simulink model "CubeSatTEST"  (R2024b)
settings: Solver=ode4  StartTime=simul.t0  StopTime=simul.tf  FixedStep=0.01  RelTol=1e-3
values from neighbouring files (symbols this model uses):
  alpha1 = 0.7    [mainSimTEST.m]
  alpha2 = 0.3    [mainSimTEST.m]
undefined symbols (not defined in the file or in its folder): act, DiscIntNeverNeededParam, env, flag, IC, K, orb, sat, sens
libraries: matrix_library x55, simulink_extras x5, simulink x2
(part 2 of 10)

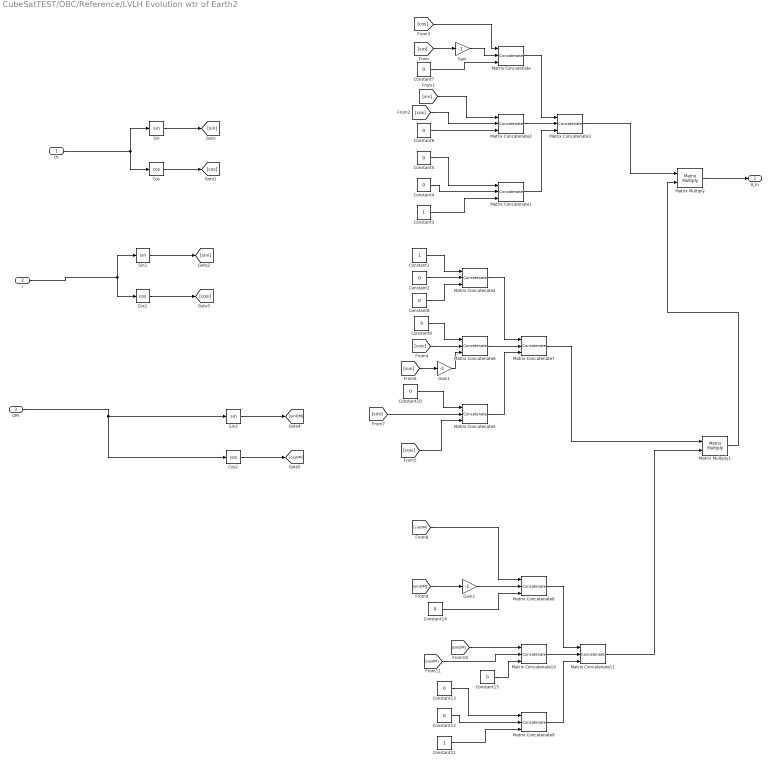
== system CubeSatTEST/OBC/Reference/LVLH Evolution wtr of Earth2 ==
  th : Inport
  i : Inport  Port=2
  OM : Inport  Port=3
  Constant1 : Constant
  Constant{2,4..10,12..15} (12 alike) : Constant  Value=0
  Constant11 : Constant
  Constant3 : Constant
  Cos : Trigonometry  Operator=cos
  Cos1 : Trigonometry  Operator=cos
  Cos2 : Trigonometry  Operator=cos
  Gain : Gain  Gain=-1
  Gain1 : Gain  Gain=-1
  Gain2 : Gain  Gain=-1
  Matrix Concatenate{,1..2,4..6,8..10} (9 alike) : Concatenate  NumInputs=3  Mode=Multidimensional array
  Matrix Concatenate11 : Concatenate  NumInputs=3  Mode=Multidimensional array  ConcatenateDimension=2
  Matrix Concatenate3 : Concatenate  NumInputs=3  Mode=Multidimensional array  ConcatenateDimension=2
  Matrix Concatenate7 : Concatenate  NumInputs=3  Mode=Multidimensional array  ConcatenateDimension=2
  Matrix Multiply : Product  Multiplication=Matrix(*)
  Matrix Multiply1 : Product  Multiplication=Matrix(*)
  Sin : Trigonometry
  Sin1 : Trigonometry
  Sin2 : Trigonometry
  A_ln : Outport
  wires:
  Cos/1 -> [cos]
  Matrix Concatenate1/1 -> Matrix Concatenate3/3
  th/1 -> Cos/1, Sin/1
  Matrix Concatenate/1 -> Matrix Concatenate3/1
  Constant5/1 -> Matrix Concatenate1/1
  Constant3/1 -> Matrix Concatenate1/3
  [cos] -> Matrix Concatenate/1
  Sin/1 -> [sin]
  Constant6/1 -> Matrix Concatenate2/3
  Constant7/1 -> Matrix Concatenate/3
  Constant4/1 -> Matrix Concatenate1/2
  Matrix Concatenate2/1 -> Matrix Concatenate3/2
  [cos] -> Matrix Concatenate2/2
  [sin] -> Matrix Concatenate2/1
  Gain/1 -> Matrix Concatenate/2
  [sin] -> Gain/1
  Cos1/1 -> [cosi]
  Sin1/1 -> [sini]
  i/1 -> Cos1/1, Sin1/1
  Matrix Multiply/1 -> A_ln/1
  Matrix Concatenate3/1 -> Matrix Multiply/1
  Matrix Concatenate6/1 -> Matrix Concatenate7/2
  Matrix Concatenate5/1 -> Matrix Concatenate7/3
  Matrix Concatenate4/1 -> Matrix Concatenate7/1
  Constant1/1 -> Matrix Concatenate4/1
  Constant2/1 -> Matrix Concatenate4/2
  Constant8/1 -> Matrix Concatenate4/3
  Constant9/1 -> Matrix Concatenate6/1
  Constant10/1 -> Matrix Concatenate5/1
  [cosi] -> Matrix Concatenate5/3
  [cosi] -> Matrix Concatenate6/2
  [sini] -> Matrix Concatenate5/2
  [sini] -> Gain1/1
  Gain1/1 -> Matrix Concatenate6/3
  Matrix Multiply1/1 -> Matrix Multiply/2
  Matrix Concatenate7/1 -> Matrix Multiply1/1
  OM/1 -> Cos2/1, Sin2/1
  Cos2/1 -> [cosOM]
  Sin2/1 -> [sinOM]
  Matrix Concatenate10/1 -> Matrix Concatenate11/2
  Matrix Concatenate9/1 -> Matrix Concatenate11/3
  Matrix Concatenate8/1 -> Matrix Concatenate11/1
  Matrix Concatenate11/1 -> Matrix Multiply1/2
  Constant13/1 -> Matrix Concatenate9/1
  Constant11/1 -> Matrix Concatenate9/3
  Constant12/1 -> Matrix Concatenate9/2
  Gain2/1 -> Matrix Concatenate8/2
  Constant14/1 -> Matrix Concatenate8/3
  [cosOM] -> Matrix Concatenate8/1
  [sinOM] -> Gain2/1
  [sinOM] -> Matrix Concatenate10/1
  [cosOM] -> Matrix Concatenate10/2
  Constant15/1 -> Matrix Concatenate10/3

== system CubeSatTEST/OBC/Reference/Magnetic Field order 1 ==
  Vector : Inport
  Clock : Clock
  Constant : Constant  Value=env.mag.dgrf2020
  Constant1 : Constant  Value=env.Earth.R
  Constant2 : Constant  Value=3
  Constant3 : Constant  Value=env.Earth.magInclination
  Constant4 : Constant  Value=3
  Cos : Trigonometry  Operator=cos
  Cos1 : Trigonometry  Operator=cos
  Divide : Product  Inputs=***/
  Divide1 : Product  Inputs=*/
  Divide2 : Product  Inputs=*/
  Dot Product : DotProduct  OutDataTypeStr=Inherit: Inherit via internal rule
  Gain : Gain  Gain=3
  Gain1 : Gain  Gain=env.Earth.omega
  Mux : Mux  Inputs=3
  Norm : Subsystem
  Norm1 : Subsystem
  Norm2 : Subsystem
  Power : Math  Operator=pow
  Power1 : Math  Operator=pow
  Product : Product
  Product1 : Product
  Product2 : Product
  Sin : Trigonometry
  Sin1 : Trigonometry
  Sqrt : Sqrt
  Square : Math  Operator=square
  Subtract : Sum  Inputs=+-
  Sum of Elements : Sum  Inputs=+
  B_n : Outport
  wires:
  Constant/1 -> Square/1
  Square/1 -> Sum of Elements/1
  Sum of Elements/1 -> Sqrt/1
  Constant1/1 -> Power/1
  Constant2/1 -> Power/2
  Sqrt/1 -> Divide/2
  Power/1 -> Divide/3
  Constant4/1 -> Power1/2
  Power1/1 -> Divide/4
  Norm/1(Norm) -> Power1/1  "norm_r"
  Vector/1 -> Norm2/1(Vector), Divide2/1, [rr]
  [rr] -> Norm/1(Vector)
  [rr_hat] -> Dot Product/2
  Subtract/1 -> Divide/1
  [mm] -> Subtract/2
  Dot Product/1 -> Product/2
  Product/1 -> Gain/1
  Gain/1 -> Subtract/1
  [rr_hat] -> Product/1
  [mm] -> Dot Product/1
  Mux/1 -> Norm1/1(Vector), Divide1/1
  Cos/1 -> Mux/3
  Constant3/1 -> Sin/1, Cos/1
  Clock/1 -> Gain1/1
  Sin/1 -> Product2/2, Product1/2
  Product1/1 -> Mux/2
  Product2/1 -> Mux/1
  Cos1/1 -> Product2/1
  Gain1/1 -> Cos1/1, Sin1/1
  Sin1/1 -> Product1/1
  Divide/1 -> B_n/1
  Norm1/1(Norm) -> Divide1/2  "norm_r"
  Divide1/1 -> [mm]
  Norm2/1(Norm) -> Divide2/2  "norm_r"
  Divide2/1 -> [rr_hat]

== system CubeSatTEST/OBC/Reference/SpaceCraft position wrt ECI1 ==
  th : Inport
  OM : Inport  Port=2
  Add : Sum
  Add1 : Sum  Inputs=+-
  Constant{1,7..10,12..15} (9 alike) : Constant  Value=0
  Constant{2..3,11,16} (4 alike) : Constant
  Constant4 : Constant  Value=2
  Constant5 : Constant  Value=orb.e
  Constant6 : Constant  Value=orb.i
  Cos{1..4} (4 alike) : Trigonometry  Operator=cos
  Divide : Product  Inputs=*/
  Gain : Gain  Gain=orb.e
  Gain1 : Gain  Gain=orb.a
  Gain2 : Gain  Gain=-1
  Gain3 : Gain  Gain=-1
  Matrix Concatenate{,4..6,8..10} (7 alike) : Concatenate  NumInputs=3  Mode=Multidimensional array
  Matrix Concatenate11 : Concatenate  NumInputs=3  Mode=Multidimensional array  ConcatenateDimension=2
  Matrix Concatenate7 : Concatenate  NumInputs=3  Mode=Multidimensional array  ConcatenateDimension=2
  Matrix Multiply : Product  Multiplication=Matrix(*)
  Matrix Multiply1 : Product  Multiplication=Matrix(*)
  Power : Math  Operator=pow
  Product2 : Product
  Sin1 : Trigonometry
  Sin2 : Trigonometry
  Sin3 : Trigonometry
  Transpose : Math  Operator=transpose
  r_n : Outport
  wires:
  Cos1/1 -> Matrix Concatenate/1
  th/1 -> Cos2/1, Sin1/1, Cos1/1
  Sin1/1 -> Matrix Concatenate/2
  Product2/1 -> r_n/1
  Divide/1 -> Product2/2
  Constant2/1 -> Add/1
  Add/1 -> Divide/2
  Cos2/1 -> Gain/1
  Gain/1 -> Add/2
  Constant3/1 -> Add1/1
  Power/1 -> Add1/2
  Constant4/1 -> Power/2
  Constant5/1 -> Power/1
  Add1/1 -> Gain1/1
  Gain1/1 -> Divide/1
  Constant6/1 -> Cos3/1, Sin2/1
  Cos3/1 -> [cosi]
  OM/1 -> Cos4/1, Sin3/1
  Sin2/1 -> [sini]
  Sin3/1 -> [sinOM]
  Cos4/1 -> [cosOM]
  Constant1/1 -> Matrix Concatenate/3
  Matrix Multiply/1 -> Product2/1
  Matrix Concatenate/1 -> Matrix Multiply/2
  Transpose/1 -> Matrix Multiply/1
  Constant15/1 -> Matrix Concatenate10/3
  [sinOM] -> Matrix Concatenate10/1
  [sinOM] -> Gain3/1
  Constant13/1 -> Matrix Concatenate9/1
  Gain2/1 -> Matrix Concatenate6/3
  Matrix Concatenate6/1 -> Matrix Concatenate7/2
  Constant14/1 -> Matrix Concatenate8/3
  [sini] -> Gain2/1
  Constant8/1 -> Matrix Concatenate4/3
  Matrix Concatenate4/1 -> Matrix Concatenate7/1
  [cosi] -> Matrix Concatenate5/3
  Constant9/1 -> Matrix Concatenate6/1
  Constant7/1 -> Matrix Concatenate4/2
  Constant10/1 -> Matrix Concatenate5/1
  Matrix Concatenate8/1 -> Matrix Concatenate11/1
  Matrix Concatenate9/1 -> Matrix Concatenate11/3
  Matrix Concatenate7/1 -> Matrix Multiply1/1
  Constant12/1 -> Matrix Concatenate9/2
  [cosi] -> Matrix Concatenate6/2
  Constant11/1 -> Matrix Concatenate9/3
  Constant16/1 -> Matrix Concatenate4/1
  [cosOM] -> Matrix Concatenate10/2
  Gain3/1 -> Matrix Concatenate8/2
  Matrix Concatenate5/1 -> Matrix Concatenate7/3
  [cosOM] -> Matrix Concatenate8/1
  Matrix Concatenate10/1 -> Matrix Concatenate11/2
  [sini] -> Matrix Concatenate5/2
  Matrix Concatenate11/1 -> Matrix Multiply1/2
  Matrix Multiply1/1 -> Transpose/1

== system CubeSatTEST/OBC/Reference/Sun Direction Circular Orbit ==
  note: Input Interface
  note: Output Interface
  Clock : Clock
  Cos : Trigonometry  Operator=cos
  Cos1 : Trigonometry  Operator=cos
  Earth's Inclination : Constant  Value=env.Earth.i
  Gain : Gain  Gain=env.Earth.n
  Matrix Concatenate : Concatenate  NumInputs=3  Mode=Multidimensional array
  Normaliser (with Built In safety) : Subsystem
  Product : Product
  Product1 : Product
  Product2 : Product
  Sin : Trigonometry
  Sin1 : Trigonometry
  Sun's Radius : Constant  Value=env.Sun.R
  S_n : Outport
  wires:
  Clock/1 -> Gain/1
  Gain/1 -> Sin/1, Cos/1
  Product/1 -> Normaliser (with Built In safety)/1(Vector)
  Sun's Radius/1 -> Product/2
  Matrix Concatenate/1 -> Product/1
  Earth's Inclination/1 -> Sin1/1, Cos1/1
  Cos1/1 -> [cos]
  Sin1/1 -> [sin]
  Cos/1 -> Matrix Concatenate/1
  Product1/1 -> Matrix Concatenate/2
  Product2/1 -> Matrix Concatenate/3
  [sin] -> Product2/2
  [cos] -> Product1/1
  Sin/1 -> Product1/2, Product2/1
  Normaliser (with Built In safety)/1(Out1) -> S_n/1

== system CubeSatTEST/Real World/DKE (Dynamics Kinematics Environment)/Dynamics ==
  note: Here we need both Newton and Euler Law
  M_ext : Inport
  Euler Integrator : Subsystem
  w_b : Outport
  wires:
  M_ext/1 -> Euler Integrator/1(M_ext)
  Euler Integrator/1(w_b) -> w_b/1

== system CubeSatTEST/Real World/DKE (Dynamics Kinematics Environment)/Environment ==
  note: This need extensive cleaning, I have no time rn
  note: Enviroment Models (Celestial Objects, Shadow, Magnetic Field, atmosphere, albedo)
  A_bn : Inport
  A_bl : Inport  Port=2
  r_n : Inport  Port=3
  Conical Shadow Model : Subsystem
  Magnetic Field order 1 : Subsystem
  Matrix Multiply : Product  Multiplication=Matrix(*)
  MatrixMultiply : Product  Multiplication=Matrix(*)
  Perturbations : Subsystem
  Scope : Scope
  Sun Direction Circular Orbit : Subsystem
  Eclipse : Outport
  S_b : Outport  Port=2
  B_b : Outport  Port=3
  Disturbance_torque : Outport  Port=4
  wires:
  Sun Direction Circular Orbit/1(S_n) -> Matrix Multiply/2, [S_n], Conical Shadow Model/1(S_n)
  Conical Shadow Model/1(eclipseFlag) -> Scope/1, Eclipse/1
  Perturbations/1(Disturbance_torque) -> Disturbance_torque/1
  r_n/1 -> Magnetic Field order 1/1(Vector), Perturbations/2(r_n), Conical Shadow Model/2(r_n)
  A_bn/1 -> Matrix Multiply/1, Perturbations/3(A_bn), MatrixMultiply/1
  [S_n] -> Perturbations/1(S_n)  "S_n"
  A_bl/1 -> Perturbations/4(A_bl)
  Matrix Multiply/1 -> S_b/1
  Magnetic Field order 1/1(Out1) -> MatrixMultiply/2
  MatrixMultiply/1 -> B_b/1

== system CubeSatTEST/Real World/DKE (Dynamics Kinematics Environment)/Kinematics ==
  note: Temp Archive
  note: B/N calculation
      | Keplerian calculations
      | L/N calculation
      | B/L calculation
  w_b : Inport
  Attitude Error : Subsystem
  Constant1 : Constant  Value=orb.i
  EulerKinematicsdelay : Subsystem
  Kepler Integrator1 : Subsystem
  Kepler Integrator2 : Subsystem  Commented=on
  LVLH Evolution wtr of Earth1 : Subsystem  Commented=on
  LVLH Evolution wtr of Earth2 : Subsystem
  SpaceCraft position wrt ECI : Subsystem
  SpaceCraft position wrt ECI1 : Subsystem  Commented=on
  A_bn : Outport
  A_bl : Outport  Port=2
  r_n : Outport  Port=3
  wires:
  w_b/1 -> EulerKinematicsdelay/1(w_b)
  Attitude Error/1(A_bl) -> A_bl/1
  EulerKinematicsdelay/1(A_bn) -> A_bn/1, Attitude Error/1(A_bn)
  LVLH Evolution wtr of Earth2/1(A_ln) -> Attitude Error/2(A_ln)
  Constant1/1 -> LVLH Evolution wtr of Earth2/2(i)
  Kepler Integrator1/1(th) -> SpaceCraft position wrt ECI/1(th), LVLH Evolution wtr of Earth2/1(th)
  SpaceCraft position wrt ECI/1(r_n) -> r_n/1
  Kepler Integrator1/2(OM) -> SpaceCraft position wrt ECI/2(OM), LVLH Evolution wtr of Earth2/3(OM)

== system CubeSatTEST/Real World/Hardware Models/Actuators ==
  note: Input Interface
  Mc_b : Inport
  w_est_b : Inport  Port=2
  w_b : Inport  Port=3
  CMG + Control Logic : Subsystem
  Constant : Constant  Value=flag.realact
  Switch : Switch  Criteria=u2 > Threshold  SaturateOnIntegerOverflow=off  InputSameDT=off
  Control_Torque_b : Outport
  vv_act_bus : Outport  Port=2
  wires:
  Constant/1 -> Switch/2
  Mc_b/1 -> [Mc_b]
  [Mc_b] -> Switch/3
  CMG + Control Logic/1(Mc) -> Switch/1
  [Mc_b] -> CMG + Control Logic/1(Mc_b)
  w_est_b/1 -> [w_est_b]
  w_b/1 -> [w_b]
  [w_est_b] -> CMG + Control Logic/2(w_mesured)
  [w_b] -> CMG + Control Logic/3(w)
  Switch/1 -> Control_Torque_b/1

== system CubeSatTEST/Real World/Hardware Models/Sensors ==
  note: Sun direction versor, MUST be normalised outside
  note: Input Interface
  note: Sun Sensors Array
  note: Output Interface
  note: Magnetometer
  S_b : Inport
  Eclipse : Inport  Port=2
  B_b : Inport  Port=3
  Bus Creator : BusCreator  Inputs=2
  Bus Creator1 : BusCreator  Inputs=2
  MAGNETOMETER : Subsystem
  SS Selector : Subsystem
  Sun Sensor (Fine) : Subsystem
  Sun Sensor (S1) : Subsystem
  Sun Sensor (S2) : Subsystem
  Sun Sensor (S3) : Subsystem
  Sun Sensor (S4) : Subsystem
  Measure : Outport
  vv_Sensor_bus : Outport  Port=2
  wires:
  Sun Sensor (S3)/1(S_meas_b) -> SS Selector/4(Course SS 3)
  Sun Sensor (Fine)/1(S_meas_b) -> SS Selector/1(Fine SS)
  Sun Sensor (S4)/1(S_meas_b) -> SS Selector/5(Course SS 4)
  Sun Sensor (S1)/1(S_meas_b) -> SS Selector/2(Course SS 1)
  Sun Sensor (S2)/1(S_meas_b) -> SS Selector/3(Course SS 2)
  S_b/1 -> [S_b]
  [S_b] -> Sun Sensor (S1)/1(S_b)
  [S_b] -> Sun Sensor (Fine)/1(S_b)
  [S_b] -> Sun Sensor (S2)/1(S_b)
  [S_b] -> Sun Sensor (S3)/1(S_b)
  [S_b] -> Sun Sensor (S4)/1(S_b)
  Eclipse/1 -> [eclipse]
  [eclipse] -> Sun Sensor (Fine)/2(eclipse)
  [eclipse] -> Sun Sensor (S1)/2(eclipse)
  [eclipse] -> Sun Sensor (S2)/2(eclipse)
  [eclipse] -> Sun Sensor (S3)/2(eclipse)
  [eclipse] -> Sun Sensor (S4)/2(eclipse)
  SS Selector/1(S_meas_b) -> [S_meas_b]
  Bus Creator/1 -> Bus Creator1/1, Measure/1  "Measure_bus"
  [S_meas_b] -> Bus Creator/1  "S_meas_b"
  [B_meas_b] -> Bus Creator/2  "B_meas_b"
  MAGNETOMETER/1(B_meas_b) -> [B_meas_b]
  B_b/1 -> [B_b]
  [B_b] -> MAGNETOMETER/1(B_b)
  SS Selector/2(vv_SS_bus) -> [vv_SS]
  Bus Creator1/1 -> vv_Sensor_bus/1  "sensor_bus"
  [vv_SS] -> Bus Creator1/2  "Sun_sensors"

== system CubeSatTEST/OBC/Guidance/Sun Pointing Guidance/Attitude Error ==
  qc : Inport
  qe : Inport  Port=2
  Matrix Multiply : Product  Multiplication=Matrix(*)
  "[q (-)]" : Subsystem
  q* : Subsystem
  dq : Outport
  wires:
  "[q (-)]"/1(Out2) -> Matrix Multiply/1
  qc/1 -> q*/1(q)
  Matrix Multiply/1 -> dq/1
  q*/1(q*) -> "[q (-)]"/1(q*)
  qe/1 -> Matrix Multiply/2

== system CubeSatTEST/OBC/Guidance/Sun Pointing Guidance/Pointing quaternion (1dof) ==
  note: Everything that enters here needs to be Normalised
  Pointing Direction : Inport
  Body Axis : Inport  Port=2
  Acos : Trigonometry  Operator=acos
  Cos : Trigonometry  Operator=cos
  Cross Product : matrix_library/Cross Product
  Demux : Demux  Outputs=3
  Dot Product : DotProduct  OutDataTypeStr=Inherit: Inherit via internal rule
  Gain : Gain  Gain=0.5
  Mux : Mux
  Product : Product
  Sin : Trigonometry
  qc : Outport
  wires:
  Mux/1 -> qc/1
  Pointing Direction/1 -> [Dir]
  Body Axis/1 -> [Body]
  [Body] -> Dot Product/1
  [Dir] -> Dot Product/2
  Dot Product/1 -> Acos/1
  Acos/1 -> Gain/1
  Gain/1 -> [O]
  [O] -> Cos/1
  Cos/1 -> Mux/4
  Demux/3 -> Mux/3
  Demux/2 -> Mux/2
  Demux/1 -> Mux/1
  Product/1 -> Demux/1
  Cross Product/1 -> Product/2
  Sin/1 -> Product/1
  [O] -> Sin/1
  [Body] -> Cross Product/1
  [Dir] -> Cross Product/2

== system CubeSatTEST/OBC/Navigation1/Angular Velocity Extimator/Xi(q) ==
  In1 : Inport
  Demux : Demux
  Gain{,1..5} (6 alike) : Gain  Gain=-1
  Matrix Concatenate : Concatenate  NumInputs=3  Mode=Multidimensional array  ConcatenateDimension=2
  Matrix Concatenate1 : Concatenate  NumInputs=4  Mode=Multidimensional array
  Matrix Concatenate2 : Concatenate  NumInputs=4  Mode=Multidimensional array
  Matrix Concatenate3 : Concatenate  NumInputs=4  Mode=Multidimensional array
  Out1 : Outport
  wires:
  In1/1 -> Demux/1
  Demux/2 -> [q2]
  Demux/3 -> [q3]
  Demux/4 -> [q4]
  Demux/1 -> [q1]
  Matrix Concatenate/1 -> Out1/1
  Matrix Concatenate1/1 -> Matrix Concatenate/1
  Matrix Concatenate2/1 -> Matrix Concatenate/2
  Matrix Concatenate3/1 -> Matrix Concatenate/3
  Gain1/1 -> Matrix Concatenate2/4
  [q1] -> Matrix Concatenate2/3
  Gain/1 -> Matrix Concatenate1/4
  [q3] -> Matrix Concatenate1/2
  [q2] -> Matrix Concatenate3/1
  Gain5/1 -> Matrix Concatenate3/4
  [q4] -> Matrix Concatenate1/1
  [q4] -> Matrix Concatenate2/2
  [q4] -> Matrix Concatenate3/3
  [q3] -> Gain2/1
  [q3] -> Gain5/1
  [q2] -> Gain3/1
  [q2] -> Gain1/1
  [q1] -> Gain/1
  [q1] -> Gain4/1
  Gain3/1 -> Matrix Concatenate1/3
  Gain2/1 -> Matrix Concatenate2/1
  Gain4/1 -> Matrix Concatenate3/2

== system CubeSatTEST/OBC/Navigation1/Angular velocity (w) computing/Q(q) ==
  q : Inport
  Demux : Demux
  Gain{1..6} (6 alike) : Gain  Gain=-1
  Matrix Concatenate : Concatenate  NumInputs=3  Mode=Multidimensional array
  Matrix Concatenate1 : Concatenate  NumInputs=4  Mode=Multidimensional array  ConcatenateDimension=2
  Matrix Concatenate2 : Concatenate  NumInputs=4  Mode=Multidimensional array  ConcatenateDimension=2
  Matrix Concatenate3 : Concatenate  NumInputs=4  Mode=Multidimensional array  ConcatenateDimension=2
  Ksi(q) : Outport
  wires:
  q/1 -> Demux/1
  Demux/2 -> [q2]
  Demux/3 -> [q3]
  Demux/4 -> [q4]
  Demux/1 -> [q1]
  Matrix Concatenate/1 -> Ksi(q)/1
  Matrix Concatenate1/1 -> Matrix Concatenate/1
  [q2] -> Matrix Concatenate2/4
  [q1] -> Matrix Concatenate2/3
  [q1] -> Matrix Concatenate1/4
  [q3] -> Matrix Concatenate1/2
  [q2] -> Gain6/1
  Gain5/1 -> Matrix Concatenate3/4
  [q4] -> Gain1/1
  [q4] -> Gain4/1
  [q4] -> Matrix Concatenate3/3
  [q3] -> Gain2/1
  [q3] -> Gain5/1
  [q2] -> Gain3/1
  Gain3/1 -> Matrix Concatenate1/3
  Gain2/1 -> Matrix Concatenate2/1
  [q1] -> Matrix Concatenate3/2
  Matrix Concatenate3/1 -> Matrix Concatenate/3
  Matrix Concatenate2/1 -> Matrix Concatenate/2
  Gain6/1 -> Matrix Concatenate3/1
  Gain4/1 -> Matrix Concatenate2/2
  Gain1/1 -> Matrix Concatenate1/1

== system CubeSatTEST/OBC/Navigation1/Angular velocity (w) computing1/Q(q) computing ==
  q1 : Inport
  q2 : Inport  Port=2
  q3 : Inport  Port=3
  q4 : Inport  Port=4
  Gain{1,3..4,7,10..11} (6 alike) : Gain  Gain=-1
  Matrix Concatenate : Concatenate  NumInputs=3  Mode=Multidimensional array
  Matrix Concatenate1 : Concatenate  NumInputs=4  Mode=Multidimensional array  ConcatenateDimension=2
  Matrix Concatenate2 : Concatenate  NumInputs=4  Mode=Multidimensional array  ConcatenateDimension=2
  Matrix Concatenate3 : Concatenate  NumInputs=4  Mode=Multidimensional array  ConcatenateDimension=2
  Q(q) : Outport
  wires:
  q1/1 -> [q1]
  q2/1 -> [q2]
  q3/1 -> [q3]
  q4/1 -> [q4]
  [q4] -> Matrix Concatenate1/1
  [q3] -> Matrix Concatenate1/2
  Gain1/1 -> Matrix Concatenate1/3
  [q2] -> Gain1/1
  Matrix Concatenate/1 -> Q(q)/1
  [q1] -> Gain3/1
  Gain3/1 -> Matrix Concatenate1/4
  [q2] -> Gain7/1
  [q1] -> Matrix Concatenate2/3
  Gain7/1 -> Matrix Concatenate2/4
  [q3] -> Gain4/1
  [q4] -> Matrix Concatenate2/2
  Gain4/1 -> Matrix Concatenate2/1
  [q3] -> Gain11/1
  [q4] -> Matrix Concatenate3/3
  [q1] -> Gain10/1
  Gain11/1 -> Matrix Concatenate3/4
  Gain10/1 -> Matrix Concatenate3/2
  [q2] -> Matrix Concatenate3/1
  Matrix Concatenate2/1 -> Matrix Concatenate/2
  Matrix Concatenate1/1 -> Matrix Concatenate/1
  Matrix Concatenate3/1 -> Matrix Concatenate/3

== system CubeSatTEST/OBC/Navigation1/Normaliser (with Built In safety)1/Norm1 ==
  Vector : Inport
  Add : Sum  Inputs=+++
  Demux : Demux  Outputs=3
  Sqrt : Sqrt
  Square : Math  Operator=square
  Square1 : Math  Operator=square
  Square2 : Math  Operator=square
  Norm : Outport
  wires:
  Square/1 -> Add/1
  Add/1 -> Sqrt/1
  Demux/3 -> Square1/1
  Square2/1 -> Add/2
  Square1/1 -> Add/3
  Demux/1 -> Square/1
  Demux/2 -> Square2/1
  Vector/1 -> Demux/1
  Sqrt/1 -> Norm/1

== system CubeSatTEST/OBC/Navigation1/Normaliser (with Built In safety)1/Protected Division ==
  Vector : Inport
  Norm : Inport  Port=2
  Constant : Constant  Value=eps
  Divide : Product  Inputs=*/
  Switch : Switch  Criteria=u2 ~= 0  SaturateOnIntegerOverflow=off  InputSameDT=off
  Out1 : Outport
  wires:
  Divide/1 -> Out1/1
  Vector/1 -> Divide/1
  Norm/1 -> Switch/1, Switch/2
  Switch/1 -> Divide/2
  Constant/1 -> Switch/3

== system CubeSatTEST/OBC/Navigation1/Normaliser (with Built In safety)2/Norm1 ==
  Vector : Inport
  Add : Sum  Inputs=+++
  Demux : Demux  Outputs=3
  Sqrt : Sqrt
  Square : Math  Operator=square
  Square1 : Math  Operator=square
  Square2 : Math  Operator=square
  Norm : Outport
  wires:
  Square/1 -> Add/1
  Add/1 -> Sqrt/1
  Demux/3 -> Square1/1
  Square2/1 -> Add/2
  Square1/1 -> Add/3
  Demux/1 -> Square/1
  Demux/2 -> Square2/1
  Vector/1 -> Demux/1
  Sqrt/1 -> Norm/1

== system CubeSatTEST/OBC/Navigation1/Normaliser (with Built In safety)2/Protected Division ==
  Vector : Inport
  Norm : Inport  Port=2
  Constant : Constant  Value=eps
  Divide : Product  Inputs=*/
  Switch : Switch  Criteria=u2 ~= 0  SaturateOnIntegerOverflow=off  InputSameDT=off
  Out1 : Outport
  wires:
  Divide/1 -> Out1/1
  Vector/1 -> Divide/1
  Norm/1 -> Switch/1, Switch/2
  Switch/1 -> Divide/2
  Constant/1 -> Switch/3

== system CubeSatTEST/OBC/Navigation1/Q method/B computing ==
  Sb : Inport
  SN : Inport  Port=2
  Bb : Inport  Port=3
  BN : Inport  Port=4
  alpha 1 : Inport  Port=5
  alpha 2 : Inport  Port=6
  Add : Sum
  Add1 : Sum
  Add2 : Sum
  Divide : Product  Inputs=*/
  Divide1 : Product  Inputs=/*
  Product : Product  Multiplication=Matrix(*)
  Product1 : Product  Multiplication=Matrix(*)
  Product2 : Product
  Product3 : Product
  Transpose : Math  Operator=transpose
  Transpose1 : Math  Operator=transpose
  B : Outport
  alpha1_normalised : Outport  Port=2
  alpha2_normalised : Outport  Port=3
  wires:
  alpha 1/1 -> [alpha_1]
  alpha 2/1 -> [alpha_2]
  [alpha_1] -> Divide/1, Add/1
  [alpha_2] -> Add/2
  Add/1 -> Divide/2
  Divide/1 -> [alpha_1_normalised]
  [alpha_2] -> Divide1/2, Add1/2
  Divide1/1 -> [alpha_2_normalised]
  [alpha_1] -> Add1/1
  Add1/1 -> Divide1/1
  SN/1 -> [SN]
  Sb/1 -> [Sb]
  Bb/1 -> [Bb]
  BN/1 -> [BN]
  Product/1 -> Add2/1
  Product1/1 -> Add2/2
  Transpose/1 -> Product/2
  [SN] -> Transpose/1
  [BN] -> Transpose1/1
  Add2/1 -> B/1
  Product2/1 -> Product/1
  [alpha_1_normalised] -> Product2/1
  [Sb] -> Product2/2
  Product3/1 -> Product1/1
  [alpha_2_normalised] -> Product3/1
  [Bb] -> Product3/2
  Transpose1/1 -> Product1/2
  [alpha_1_normalised] -> alpha1_normalised/1
  [alpha_2_normalised] -> alpha2_normalised/1

== system CubeSatTEST/OBC/Navigation1/Q method/S and Z matrix computing ==
  B : Inport
  Add : Sum
  Add1 : Sum  Inputs=+-
  Add2 : Sum  Inputs=+-
  Add3 : Sum  Inputs=+-
  Add4 : Sum  Commented=on  Inputs=+-
  From1 : From  Commented=on  GotoTag=B
  From3 : From  Commented=on  GotoTag=Z
  From4 : From  Commented=on  GotoTag=Sigma
  From5 : From  Commented=on  GotoTag=S
  From6 : From  Commented=on  GotoTag=Z
  From7 : From  Commented=on  GotoTag=Sigma
  Goto2 : Goto  Commented=on  GotoTag=Sigma
  IdentityMatrix : IdentityMatrix  Commented=on
  Matrix Concatenate : Concatenate  Commented=on  NumInputs=4  Mode=Multidimensional array  ConcatenateDimension=2
  Mux : Mux  Inputs=3
  Product : Product  Commented=on
  Selector : Selector  NumberOfDimensions=2  InputPortWidth=3  IndexOptions=Index vector (dialog),Index vector (dialog)  Indices=2,3  OutputSizes=1,1
  Selector1 : Selector  NumberOfDimensions=2  InputPortWidth=3  IndexOptions=Index vector (dialog),Index vector (dialog)  Indices=3,2  OutputSizes=1,1
  Selector2 : Selector  NumberOfDimensions=2  InputPortWidth=3  IndexOptions=Index vector (dialog),Index vector (dialog)  Indices=3,1  OutputSizes=1,1
  Selector3 : Selector  NumberOfDimensions=2  InputPortWidth=3  IndexOptions=Index vector (dialog),Index vector (dialog)  Indices=1,3  OutputSizes=1,1
  Selector4 : Selector  NumberOfDimensions=2  InputPortWidth=3  IndexOptions=Index vector (dialog),Index vector (dialog)  Indices=1,2  OutputSizes=1,1
  Selector5 : Selector  NumberOfDimensions=2  InputPortWidth=3  IndexOptions=Index vector (dialog),Index vector (dialog)  Indices=2,1  OutputSizes=1,1
  Trace : Subsystem  Commented=on
  Transpose : matrix_library/Transpose
  Transpose1 : matrix_library/Transpose  Commented=on
  S : Outport
  Z : Outport  Port=2
  wires:
  [B] -> Add/1, Transpose/1
  Transpose/1 -> Add/2
  Add/1 -> [S]
  B/1 -> [B]
  From1/1 -> Trace/1(In1)
  Trace/1(Out1) -> Goto2/1
  [B] -> Selector/1, Selector1/1, Selector2/1, Selector5/1, Selector4/1, Selector3/1
  Selector/1 -> Add1/1
  Selector1/1 -> Add1/2
  Selector4/1 -> Add3/1
  Selector5/1 -> Add3/2
  Selector3/1 -> Add2/2
  Selector2/1 -> Add2/1
  Add1/1 -> Mux/1
  Add2/1 -> Mux/2
  Add3/1 -> Mux/3
  Mux/1 -> [Z]
  From3/1 -> Matrix Concatenate/2
  From4/1 -> Product/1
  IdentityMatrix/1 -> Product/2
  Product/1 -> Add4/2
  From5/1 -> Add4/1
  Add4/1 -> Matrix Concatenate/1
  Transpose1/1 -> Matrix Concatenate/3
  From6/1 -> Transpose1/1
  From7/1 -> Matrix Concatenate/4
  [S] -> S/1
  [Z] -> Z/1

== system CubeSatTEST/OBC/Navigation1/Q method/Subsystem ==
  alpha2_normalised : Inport
  alpha1_normalised : Inport  Port=2
  B_b : Inport  Port=3
  B_N : Inport  Port=4
  S_b : Inport  Port=5
  S_N : Inport  Port=6
  Add : Sum
  Add1 : Sum
  Add2 : Sum
  Constant : Constant  Value=2
  Cross Product : matrix_library/Cross Product
  Cross Product1 : matrix_library/Cross Product
  Dot Product : DotProduct  OutDataTypeStr=Inherit: Inherit via internal rule
  Dot Product1 : DotProduct  OutDataTypeStr=Inherit: Inherit via internal rule
  From16 : From
  Goto12 : Goto
  Math Function : Math  Operator=square
  Math Function1 : Math  Operator=square
  Norm1 : Subsystem
  Norm2 : Subsystem
  Product : Product
  Product1 : Product
  Product2 : Product
  Product3 : Product  Inputs=3
  Sqrt : Sqrt
  lambda_max : Outport
  wires:
  Math Function/1 -> Add/1
  Math Function1/1 -> Add/2
  Dot Product/1 -> [dotb1b2]
  Dot Product1/1 -> [dotr1r2]
  [dotr1r2] -> Product/2
  [dotb1b2] -> Product/1
  B_b/1 -> [Bb]
  S_b/1 -> [Sb]
  B_N/1 -> [BN]
  S_N/1 -> [SN]
  [Sb] -> Dot Product/2
  [Bb] -> Dot Product/1
  [SN] -> Dot Product1/2
  [Bb] -> Cross Product1/1
  [Sb] -> Cross Product1/2
  [BN] -> Cross Product/1
  [SN] -> Cross Product/2
  Cross Product1/1 -> Norm1/1(Vector)
  Cross Product/1 -> Norm2/1(Vector)
  [crossb1b2] -> Product1/1
  [crossr1r2] -> Product1/2
  Product1/1 -> Add1/2
  Product/1 -> Add1/1
  alpha2_normalised/1 -> [alpha2_normalised]
  alpha1_normalised/1 -> [alpha1_normalised]
  [alpha1_normalised] -> Math Function/1
  [alpha2_normalised] -> Math Function1/1
  [alpha2_normalised] -> Product3/3
  [alpha1_normalised] -> Product3/2
  Constant/1 -> Product3/1
  Add1/1 -> [C]
  Product3/1 -> [B]
  Add/1 -> Goto12/1
  From16/1 -> Add2/1
  Add2/1 -> Sqrt/1
  Sqrt/1 -> lambda_max/1
  [BN] -> Dot Product1/1
  Norm1/1(Norm) -> [crossb1b2]  "norm_r"
  Norm2/1(Norm) -> [crossr1r2]  "norm_r"
  Product2/1 -> Add2/2
  [B] -> Product2/1
  [C] -> Product2/2

== system CubeSatTEST/OBC/Navigation1/Q method/q_opt computing ==
  S : Inport
  Z : Inport  Port=2
  lambda_max : Inport  Port=3
  B : Inport  Port=4
  Add : Sum
  Add1 : Sum  Inputs=+-
  Adj 3x3 : Subsystem
  Det 3x3 : Subsystem
  Divide : Product  Inputs=*/
  IdentityMatrix : IdentityMatrix  OutputDimensions=3
  Matrix Concatenate : Concatenate  Mode=Multidimensional array
  Product : Product
  Product1 : Product  Multiplication=Matrix(*)
  Scope : Scope
  Trace : Subsystem
  ||q||1 : Subsystem
  q_opt : Outport
  wires:
  B/1 -> Trace/1(B)
  lambda_max/1 -> Add/2
  Trace/1(tr(B)) -> Add/1
  Add/1 -> [p]
  IdentityMatrix/1 -> Product/2
  [p] -> Product/1
  Product/1 -> [pI3]
  S/1 -> Add1/2
  [pI3] -> Add1/1
  Add1/1 -> Det 3x3/1(A), Adj 3x3/1(A)
  Matrix Concatenate/1 -> [q]
  [q] -> Divide/1
  Divide/1 -> q_opt/1
  Z/1 -> Product1/2
  Product1/1 -> Matrix Concatenate/1
  ||q||1/1(Out1) -> Divide/2
  [q] -> ||q||1/1(q)
  Adj 3x3/1(Adj(A)) -> Product1/1
  Det 3x3/1(det(A)) -> Scope/1, Matrix Concatenate/2

== system CubeSatTEST/OBC/Navigation1/Sequential Rotations/If Action Subsystem ==
  Sn : Inport
  Bn : Inport  Port=2
  Action Port : ActionPort  ActionPortLabel=else
  Out1 : Outport
  Out2 : Outport  Port=2
  wires:
  Sn/1 -> Out1/1
  Bn/1 -> Out2/1

== system CubeSatTEST/OBC/Navigation1/Sequential Rotations/If Action Subsystem1 ==
  q_estimated : Inport
  Action Port : ActionPort  ActionPortLabel=else
  Out1 : Outport
  wires:
  q_estimated/1 -> Out1/1

== system CubeSatTEST/OBC/Navigation1/Sequential Rotations/If Action Subsystem2 ==
  Sn : Inport
  Bn : Inport  Port=2
  flag : Inport  Port=3
  Action Port : ActionPort  ActionPortLabel=if(u1 < 0)
  Abs : Abs  SaturateOnIntegerOverflow=off
  Demux : Demux
  Demux1 : Demux
  If : If  NumInputs=3  IfExpression="(u3 >= u1)  & (u3>=u2)"  ElseIfExpressions=(u2>=u1) & (u2>=u3)
  If1 : If  NumInputs=3  IfExpression="(u3 >= u1)  & (u3>=u2)"  ElseIfExpressions=(u2>=u1) & (u2>=u3)
  Merge : Merge  Inputs=3
  Merge1 : Merge  Inputs=3
  Reference Rotator x : Subsystem
  Reference Rotator x1 : Subsystem
  Reference Rotator y : Subsystem
  Reference Rotator y1 : Subsystem
  Reference Rotator z : Subsystem
  Reference Rotator z1 : Subsystem
  Terminator : Terminator
  Terminator1 : Terminator
  S_n' : Outport
  B_n' : Outport  Port=2
  wires:
  Demux/1 -> If/1
  Demux/4 -> Terminator/1
  Demux/2 -> If/2
  Demux/3 -> If/3
  Demux1/3 -> If1/3
  Demux1/2 -> If1/2
  Demux1/1 -> If1/1
  Demux1/4 -> Terminator1/1
  Reference Rotator y/1(Out1) -> Merge/2
  Reference Rotator x/1(Out1) -> Merge/1
  Reference Rotator z/1(Out1) -> Merge/3
  If/3 -> Reference Rotator x/Action
  If/2 -> Reference Rotator y/Action
  If/1 -> Reference Rotator z/Action
  Sn/1 -> Reference Rotator y/1(S_N), Reference Rotator x/1(S_N), Reference Rotator z/1(S_N)
  Reference Rotator y1/1(Out1) -> Merge1/2
  Reference Rotator z1/1(Out1) -> Merge1/3
  Reference Rotator x1/1(Out1) -> Merge1/1
  If1/1 -> Reference Rotator z1/Action
  If1/2 -> Reference Rotator y1/Action
  If1/3 -> Reference Rotator x1/Action
  Bn/1 -> Reference Rotator z1/1(S_N), Reference Rotator y1/1(S_N), Reference Rotator x1/1(S_N)
  flag/1 -> Abs/1
  Merge/1 -> S_n'/1
  Merge1/1 -> B_n'/1
  Abs/1 -> Demux/1, Demux1/1

== system CubeSatTEST/OBC/Navigation1/Sequential Rotations/If Action Subsystem3 ==
  q_estimated : Inport
  flag : Inport  Port=2
  Action Port : ActionPort  ActionPortLabel=if(u1 < 0)
  Abs : Abs  SaturateOnIntegerOverflow=off
  Attitude Recovery x : Subsystem
  Attitude Recovery y : Subsystem
  Attitude Recovery z : Subsystem
  Demux : Demux
  If : If  NumInputs=3  IfExpression="(u3 >= u1)  & (u3>=u2)"  ElseIfExpressions=(u2>=u1) & (u2>=u3)
  Merge : Merge  Inputs=3
  Terminator : Terminator
  Out1 : Outport
  wires:
  Demux/1 -> If/1
  Demux/2 -> If/2
  Demux/3 -> If/3
  Demux/4 -> Terminator/1
  Attitude Recovery z/1(Out1) -> Merge/1
  Attitude Recovery y/1(Out1) -> Merge/2
  Attitude Recovery x/1(Out1) -> Merge/3
  If/1 -> Attitude Recovery z/Action
  If/2 -> Attitude Recovery y/Action
  If/3 -> Attitude Recovery x/Action
  q_estimated/1 -> [q]
  [q] -> Attitude Recovery z/1(q_estimated)
  [q] -> Attitude Recovery y/1(q_estimated)
  [q] -> Attitude Recovery x/1(q_estimated)
  flag/1 -> Abs/1
  Merge/1 -> Out1/1
  Abs/1 -> Demux/1

== system CubeSatTEST/OBC/Navigation1/Sequential Rotations/Q method ==
  S_b : Inport
  B_b : Inport  Port=2
  S_N : Inport  Port=3
  B_N : Inport  Port=4
  alpha 1 : Inport  Port=5
  alpha 2 : Inport  Port=6
  B computing : Subsystem
      settings: PortSchema="{\"entries\":[{\"content\":{\"sides\":[{\"content\":{\"connectorIds\":[\"In1\",\"In2\",\"In3\",\"In4\"]},\"type\":\"ConnectorPlacement.EquallySpacedRectSide\",\"uuid\":\"50fc9399-82b5-4b10-921b-f93011029ce3\"},{\"content\":{\"connectorIds\":[\"Out1\"],\"side\":\"RIGHT\"},\"type\":\"ConnectorPlacement.EquallySpacedRectSide\",\"uuid\":\"3981c554-ab38-4f62-9b84-94877d1cd2ff\"},{\"content\":{\"connectorIds\":[\"Out2\",\"Out3\"],\"side\":\"TOP\"},\"type\":\"ConnectorPlacement.EquallySpacedRectSide\",\"uuid\":\"ba062d99-6f44-4068-8114-c0cfa81f1ff2\"},{\"content\":{\"connectorIds\":[\"In5\",\"In6\"],\"side\":\"BOTTOM\"},\"type\":\"ConnectorPlacement.EquallySpacedRectSide\",\"uuid\":\"0ce0d8e8-da8b-4b2d-90df-7b0bc851bc5b\"}]},\"type\":\"ConnectorPlacement.EquallySpacedConnector\",\"uuid\":\"bcda7430-c6c8-4f59-a99a-b367d20ffcb5\"}],\"packageUris\":[\"http://schema.mathworks.com/mf0/Connector/R2020b\"],\"version\":\"1.0\"}"
  S and Z matrix computing : Subsystem
  Scope : Scope
  Subsystem : Subsystem
      settings: PortSchema="{\"entries\":[{\"content\":{\"sides\":[{\"content\":{\"connectorIds\":[\"Out1\"]},\"type\":\"ConnectorPlacement.EquallySpacedRectSide\",\"uuid\":\"5768cb62-7f28-4cce-8da1-dcdd14add895\"},{\"content\":{\"side\":\"RIGHT\"},\"type\":\"ConnectorPlacement.EquallySpacedRectSide\",\"uuid\":\"8778aa17-5802-4f6c-9df9-b85455c7c074\"},{\"content\":{\"connectorIds\":[\"In1\",\"In2\"],\"side\":\"TOP\"},\"type\":\"ConnectorPlacement.EquallySpacedRectSide\",\"uuid\":\"8a3cb844-269f-4d3f-b8ee-2af4584390c1\"},{\"content\":{\"connectorIds\":[\"In3\",\"In4\",\"In5\",\"In6\"],\"side\":\"BOTTOM\"},\"type\":\"ConnectorPlacement.EquallySpacedRectSide\",\"uuid\":\"ccc3bad4-265e-44f4-a8b0-aae769a28e60\"}]},\"type\":\"ConnectorPlacement.EquallySpacedConnector\",\"uuid\":\"9389ccda-4d08-49a8-9951-bd9019203c57\"}],\"packageUris\":[\"http://schema.mathworks.com/mf0/Connector/R2020b\"],\"version\":\"1.0\"}"
  q_opt computing : Subsystem
      settings: PortSchema="{\"entries\":[{\"content\":{\"sides\":[{\"content\":{\"connectorIds\":[\"In1\",\"In2\"]},\"type\":\"ConnectorPlacement.EquallySpacedRectSide\",\"uuid\":\"077e0174-8a2c-4f76-bac9-e91df836f5e1\"},{\"content\":{\"connectorIds\":[\"Out1\",\"In4\"],\"side\":\"RIGHT\"},\"type\":\"ConnectorPlacement.EquallySpacedRectSide\",\"uuid\":\"0e923535-8f32-4607-bd4a-42896d211835\"},{\"content\":{\"connectorIds\":[\"In3\"],\"side\":\"TOP\"},\"type\":\"ConnectorPlacement.EquallySpacedRectSide\",\"uuid\":\"91682e2a-1ae8-44b6-9458-d5d75f2c9b10\"},{\"content\":{\"side\":\"BOTTOM\"},\"type\":\"ConnectorPlacement.EquallySpacedRectSide\",\"uuid\":\"ebee2d10-c6a3-420b-a3da-5d4d259a0e4d\"}]},\"type\":\"ConnectorPlacement.EquallySpacedConnector\",\"uuid\":\"6651e596-192f-4f32-9855-13a8c081df01\"}],\"packageUris\":[\"http://schema.mathworks.com/mf0/Connector/R2020b\"],\"version\":\"1.0\"}"
  q_estimated : Outport
  wires:
  alpha 1/1 -> [alpha1]
  [B_b] -> B computing/3(Bb)
  S_b/1 -> [S_b]
  [B_N] -> B computing/4(BN)
  [S_N] -> B computing/2(SN)
  B computing/1(B) -> q_opt computing/4(B), S and Z matrix computing/1(B)
  [S_N] -> Subsystem/6(S_N)
  [B_b] -> Subsystem/3(B_b)
  [S_b] -> Subsystem/5(S_b)
  B_N/1 -> [B_N]
  S_N/1 -> [S_N]
  B_b/1 -> [B_b]
  [alpha1] -> B computing/5(alpha 1)
  [S_b] -> B computing/1(Sb)
  S and Z matrix computing/1(S) -> q_opt computing/1(S)
  [alpha2] -> B computing/6(alpha 2)
  alpha 2/1 -> [alpha2]
  S and Z matrix computing/2(Z) -> q_opt computing/2(Z)
  q_opt computing/1(q_opt) -> q_estimated/1
  [B_N] -> Subsystem/4(B_N)
  B computing/2(alpha1_normalised) -> Subsystem/2(alpha1_normalised)
  B computing/3(alpha2_normalised) -> Subsystem/1(alpha2_normalised)
  Subsystem/1(lambda_max) -> Scope/1, q_opt computing/3(lambda_max)

== system CubeSatTEST/OBC/Navigation1/Sequential Rotations + Q method/If Action Subsystem1 ==
  q_estimated : Inport
  Action Port : ActionPort  ActionPortLabel=if(u1 < 0.2)
  Out1 : Outport
  wires:
  q_estimated/1 -> Out1/1

== system CubeSatTEST/OBC/Navigation1/Sequential Rotations + Q method/Q method ==
  S_b : Inport
  B_b : Inport  Port=2
  S_N : Inport  Port=3
  B_N : Inport  Port=4
  alpha 1 : Inport  Port=5
  alpha 2 : Inport  Port=6
  B computing : Subsystem
      settings: PortSchema="{\"entries\":[{\"content\":{\"sides\":[{\"content\":{\"connectorIds\":[\"In1\",\"In2\",\"In3\",\"In4\"]},\"type\":\"ConnectorPlacement.EquallySpacedRectSide\",\"uuid\":\"50fc9399-82b5-4b10-921b-f93011029ce3\"},{\"content\":{\"connectorIds\":[\"Out1\"],\"side\":\"RIGHT\"},\"type\":\"ConnectorPlacement.EquallySpacedRectSide\",\"uuid\":\"3981c554-ab38-4f62-9b84-94877d1cd2ff\"},{\"content\":{\"connectorIds\":[\"Out2\",\"Out3\"],\"side\":\"TOP\"},\"type\":\"ConnectorPlacement.EquallySpacedRectSide\",\"uuid\":\"ba062d99-6f44-4068-8114-c0cfa81f1ff2\"},{\"content\":{\"connectorIds\":[\"In5\",\"In6\"],\"side\":\"BOTTOM\"},\"type\":\"ConnectorPlacement.EquallySpacedRectSide\",\"uuid\":\"0ce0d8e8-da8b-4b2d-90df-7b0bc851bc5b\"}]},\"type\":\"ConnectorPlacement.EquallySpacedConnector\",\"uuid\":\"bcda7430-c6c8-4f59-a99a-b367d20ffcb5\"}],\"packageUris\":[\"http://schema.mathworks.com/mf0/Connector/R2020b\"],\"version\":\"1.0\"}"
  S and Z matrix computing : Subsystem
  Scope : Scope
  Scope1 : Scope
  Scope2 : Scope
  Subsystem : Subsystem
      settings: PortSchema="{\"entries\":[{\"content\":{\"sides\":[{\"content\":{\"connectorIds\":[\"Out1\"]},\"type\":\"ConnectorPlacement.EquallySpacedRectSide\",\"uuid\":\"5768cb62-7f28-4cce-8da1-dcdd14add895\"},{\"content\":{\"side\":\"RIGHT\"},\"type\":\"ConnectorPlacement.EquallySpacedRectSide\",\"uuid\":\"8778aa17-5802-4f6c-9df9-b85455c7c074\"},{\"content\":{\"connectorIds\":[\"In1\",\"In2\"],\"side\":\"TOP\"},\"type\":\"ConnectorPlacement.EquallySpacedRectSide\",\"uuid\":\"8a3cb844-269f-4d3f-b8ee-2af4584390c1\"},{\"content\":{\"connectorIds\":[\"In3\",\"In4\",\"In5\",\"In6\"],\"side\":\"BOTTOM\"},\"type\":\"ConnectorPlacement.EquallySpacedRectSide\",\"uuid\":\"ccc3bad4-265e-44f4-a8b0-aae769a28e60\"}]},\"type\":\"ConnectorPlacement.EquallySpacedConnector\",\"uuid\":\"9389ccda-4d08-49a8-9951-bd9019203c57\"}],\"packageUris\":[\"http://schema.mathworks.com/mf0/Connector/R2020b\"],\"version\":\"1.0\"}"
  q_opt computing : Subsystem
      settings: PortSchema="{\"entries\":[{\"content\":{\"sides\":[{\"content\":{\"connectorIds\":[\"In1\",\"In2\"]},\"type\":\"ConnectorPlacement.EquallySpacedRectSide\",\"uuid\":\"077e0174-8a2c-4f76-bac9-e91df836f5e1\"},{\"content\":{\"connectorIds\":[\"Out1\",\"In4\"],\"side\":\"RIGHT\"},\"type\":\"ConnectorPlacement.EquallySpacedRectSide\",\"uuid\":\"0e923535-8f32-4607-bd4a-42896d211835\"},{\"content\":{\"connectorIds\":[\"In3\"],\"side\":\"TOP\"},\"type\":\"ConnectorPlacement.EquallySpacedRectSide\",\"uuid\":\"91682e2a-1ae8-44b6-9458-d5d75f2c9b10\"},{\"content\":{\"side\":\"BOTTOM\"},\"type\":\"ConnectorPlacement.EquallySpacedRectSide\",\"uuid\":\"ebee2d10-c6a3-420b-a3da-5d4d259a0e4d\"}]},\"type\":\"ConnectorPlacement.EquallySpacedConnector\",\"uuid\":\"6651e596-192f-4f32-9855-13a8c081df01\"}],\"packageUris\":[\"http://schema.mathworks.com/mf0/Connector/R2020b\"],\"version\":\"1.0\"}"
  q_estimated : Outport
  wires:
  alpha 1/1 -> [alpha1]
  [B_b] -> B computing/3(Bb)
  S_b/1 -> [S_b]
  [B_N] -> B computing/4(BN)
  [S_N] -> B computing/2(SN)
  B computing/1(B) -> q_opt computing/4(B), S and Z matrix computing/1(B)
  [S_N] -> Subsystem/6(S_N)
  [B_b] -> Subsystem/3(B_b)
  [S_b] -> Subsystem/5(S_b)
  B_N/1 -> [B_N]
  S_N/1 -> [S_N]
  B_b/1 -> [B_b]
  [alpha1] -> B computing/5(alpha 1)
  [S_b] -> B computing/1(Sb)
  S and Z matrix computing/1(S) -> Scope1/1, q_opt computing/1(S)
  [alpha2] -> B computing/6(alpha 2)
  alpha 2/1 -> [alpha2]
  S and Z matrix computing/2(Z) -> Scope2/1, q_opt computing/2(Z)
  q_opt computing/1(q_opt) -> q_estimated/1
  [B_N] -> Subsystem/4(B_N)
  B computing/2(alpha1_normalised) -> Subsystem/2(alpha1_normalised)
  B computing/3(alpha2_normalised) -> Subsystem/1(alpha2_normalised)
  Subsystem/1(lambda_max) -> Scope/1, q_opt computing/3(lambda_max)

== system CubeSatTEST/OBC/Navigation1/Sequential Rotations + Q method/Reference Rotator z ==
  S_N : Inport
  Demux : Demux  Outputs=3
  Gain : Gain  Gain=-1
  Gain1 : Gain
  Gain2 : Gain  Gain=-1
  Mux : Mux  Inputs=3
  B_N : Outport
  wires:
  Gain2/1 -> Mux/1
  Gain/1 -> Mux/2
  Mux/1 -> B_N/1
  Gain1/1 -> Mux/3
  S_N/1 -> Demux/1
  Demux/1 -> Gain2/1
  Demux/2 -> Gain/1
  Demux/3 -> Gain1/1

== system CubeSatTEST/OBC/Navigation1/Sequential Rotations + Q method/Reference Rotator z1 ==
  S_N : Inport
  Demux : Demux  Outputs=3
  Gain : Gain  Gain=-1
  Gain1 : Gain
  Gain2 : Gain  Gain=-1
  Mux : Mux  Inputs=3
  Out1 : Outport
  wires:
  Gain2/1 -> Mux/1
  Gain/1 -> Mux/2
  Mux/1 -> Out1/1
  Gain1/1 -> Mux/3
  S_N/1 -> Demux/1
  Demux/1 -> Gain2/1
  Demux/2 -> Gain/1
  Demux/3 -> Gain1/1

== system CubeSatTEST/OBC/Navigation1/Sequential Rotations + Q method/Z ==
  q_estimated : Inport
  flag : Inport  Port=2
  S_b : Inport  Port=3
  B_b : Inport  Port=4
  S_Nr : Inport  Port=5
  B_Nr : Inport  Port=6
  S_n : Inport  Port=7
  B_n : Inport  Port=8
  Action Port : ActionPort  ActionPortLabel=else
  Abs1 : Abs  SaturateOnIntegerOverflow=off
  If Action Subsystem1 : Subsystem  TreatAsAtomicUnit=on
  If1 : If  IfExpression=u1 < 0.2
  Merge1 : Merge
  Q method z : Subsystem
      settings: PortSchema="{\"entries\":[{\"content\":{\"sides\":[{\"content\":{\"connectorIds\":[\"In1\",\"In2\",\"In3\",\"In4\"]},\"type\":\"ConnectorPlacement.EquallySpacedRectSide\",\"uuid\":\"15956c10-3c30-4cb4-a63c-f434daa5cd48\"},{\"content\":{\"connectorIds\":[\"Out1\"],\"side\":\"RIGHT\"},\"type\":\"ConnectorPlacement.EquallySpacedRectSide\",\"uuid\":\"3f26d307-35c8-43a0-9998-86e1286678fb\"},{\"content\":{\"connectorIds\":[\"In5\",\"In6\"],\"side\":\"TOP\"},\"type\":\"ConnectorPlacement.EquallySpacedRectSide\",\"uuid\":\"55f51305-766e-4e3f-8617-95c7676083b2\"}]},\"type\":\"ConnectorPlacement.EquallySpacedConnector\",\"uuid\":\"09b6cbb7-0430-4316-92af-7ec4423129aa\"}],\"packageUris\":[\"http://schema.mathworks.com/mf0/Connector/R2020b\"],\"version\":\"1.0\"}"
  Reference Rotator y : Subsystem
  Reference Rotator y1 : Subsystem
  Selector1 : Selector  InputPortWidth=4  IndexOptions=Index vector (dialog)  Indices=4  OutputSizes=1
  Y : Subsystem  TreatAsAtomicUnit=on
  Out1 : Outport
  wires:
  S_Nr/1 -> Q method z/3(S_N)
  If1/1 -> If Action Subsystem1/Action
  Selector1/1 -> Abs1/1
  Abs1/1 -> If1/1
  Merge1/1 -> Out1/1
  If1/2 -> Y/Action
  B_Nr/1 -> Q method z/4(B_N)
  S_b/1 -> Y/3(S_b), Q method z/1(S_b)
  Q method z/1(q_estimated) -> If Action Subsystem1/1(q_estimated), [flag]
  B_b/1 -> Y/4(B_b), Q method z/2(B_b)
  Y/1(Out1) -> Merge1/2
  [flag] -> Selector1/1
  If Action Subsystem1/1(Out1) -> Merge1/1
  [alpha2] -> Q method z/6(alpha 2)
  flag/1 -> [alpha2]
  [alpha1] -> Q method z/5(alpha 1)
  q_estimated/1 -> [alpha1]
  [alpha2] -> Y/2(flag)
  [alpha1] -> Y/1(q_estimated)
  Reference Rotator y/1(B_N) -> Y/6(B_Nr)
  Reference Rotator y1/1(Out1) -> Y/5(S_Nr)
  S_n/1 -> Y/7(S_n), Reference Rotator y1/1(S_N)
  B_n/1 -> Y/8(B_n), Reference Rotator y/1(S_N)

== system CubeSatTEST/OBC/Navigation1/Sequential Rotations Playground/Enable second check ==
  Action Port : ActionPort  ActionPortLabel=else
  Constant : Constant
  Out1 : Outport
  wires:
  Constant/1 -> Out1/1

== system CubeSatTEST/OBC/Navigation1/Sequential Rotations Playground/Enable second check1 ==
  Action Port : ActionPort  ActionPortLabel=else
  Constant : Constant
  Out1 : Outport
  wires:
  Constant/1 -> Out1/1

== system CubeSatTEST/OBC/Navigation1/Sequential Rotations Playground/Max ==
  In1 : Inport
  q : Inport  Port=2
  Abs : Abs  SaturateOnIntegerOverflow=off
  Attitude Recovery x : Subsystem
  Attitude Recovery y : Subsystem
  Attitude Recovery z : Subsystem
  Constant : Constant  Value=[1; 1; 1; 1]
  Demux : Demux
  Enable second check : Subsystem  TreatAsAtomicUnit=on
  If : If  NumInputs=2  IfExpression=(u1 == 0)  ElseIfExpressions=(u2 == 0)
  If1 : If  NumInputs=3  IfExpression=(u1 == 1)&(u2==0)  ElseIfExpressions=(u1 == 1)&(u3==0)  ShowElse=off
  Max of Elements : MinMax  Function=max
  Merge : Merge  Inputs=4
  Product : Product
  Subtract : Sum  Inputs=-+
  Switch Case Action Subsystem2 : Subsystem  TreatAsAtomicUnit=on
  Index : Outport
  wires:
  If/1 -> Switch Case Action Subsystem2/Action
  Demux/3 -> [q3]
  If1/2 -> Attitude Recovery x/Action
  [q4] -> If/1
  [q1] -> If1/3
  Constant/1 -> Product/1
  Enable second check/1(Out1) -> If1/1
  If/2 -> Attitude Recovery z/Action
  Max of Elements/1 -> Product/2
  If/3 -> Enable second check/Action
  Subtract/1 -> Abs/1
  Demux/2 -> [q2]
  Product/1 -> Subtract/1
  Demux/1 -> [q1]
  Demux/4 -> [q4]
  [q3] -> If/2
  [q2] -> If1/2
  Switch Case Action Subsystem2/1(Out1) -> Merge/1
  If1/1 -> Attitude Recovery y/Action
  Merge/1 -> Index/1
  Attitude Recovery y/1(Out1) -> Merge/3
  Attitude Recovery x/1(Out1) -> Merge/4
  [q] -> Switch Case Action Subsystem2/1(S_N)
  [q] -> Attitude Recovery z/1(q_estimated)
  Attitude Recovery z/1(Out1) -> Merge/2
  [q] -> Attitude Recovery y/1(q_estimated)
  [q] -> Attitude Recovery x/1(q_estimated)
  q/1 -> [q]
  In1/1 -> Subtract/2, Max of Elements/1
  Abs/1 -> Demux/1

== system CubeSatTEST/OBC/Navigation1/Sequential Rotations Playground/Q method ==
  S_b : Inport
  S_N : Inport  Port=2
  B_b : Inport  Port=3
  B_N : Inport  Port=4
  alpha 1 : Inport  Port=5
  alpha 2 : Inport  Port=6
  B computing : Subsystem
      settings: PortSchema="{\"entries\":[{\"content\":{\"sides\":[{\"content\":{\"connectorIds\":[\"In1\",\"In2\",\"In3\",\"In4\"]},\"type\":\"ConnectorPlacement.EquallySpacedRectSide\",\"uuid\":\"50fc9399-82b5-4b10-921b-f93011029ce3\"},{\"content\":{\"connectorIds\":[\"Out1\"],\"side\":\"RIGHT\"},\"type\":\"ConnectorPlacement.EquallySpacedRectSide\",\"uuid\":\"3981c554-ab38-4f62-9b84-94877d1cd2ff\"},{\"content\":{\"connectorIds\":[\"Out2\",\"Out3\"],\"side\":\"TOP\"},\"type\":\"ConnectorPlacement.EquallySpacedRectSide\",\"uuid\":\"ba062d99-6f44-4068-8114-c0cfa81f1ff2\"},{\"content\":{\"connectorIds\":[\"In5\",\"In6\"],\"side\":\"BOTTOM\"},\"type\":\"ConnectorPlacement.EquallySpacedRectSide\",\"uuid\":\"0ce0d8e8-da8b-4b2d-90df-7b0bc851bc5b\"}]},\"type\":\"ConnectorPlacement.EquallySpacedConnector\",\"uuid\":\"bcda7430-c6c8-4f59-a99a-b367d20ffcb5\"}],\"packageUris\":[\"http://schema.mathworks.com/mf0/Connector/R2020b\"],\"version\":\"1.0\"}"
  S and Z matrix computing : Subsystem
  Scope : Scope
  Subsystem : Subsystem
      settings: PortSchema="{\"entries\":[{\"content\":{\"sides\":[{\"content\":{\"connectorIds\":[\"Out1\"]},\"type\":\"ConnectorPlacement.EquallySpacedRectSide\",\"uuid\":\"5768cb62-7f28-4cce-8da1-dcdd14add895\"},{\"content\":{\"side\":\"RIGHT\"},\"type\":\"ConnectorPlacement.EquallySpacedRectSide\",\"uuid\":\"8778aa17-5802-4f6c-9df9-b85455c7c074\"},{\"content\":{\"connectorIds\":[\"In1\",\"In2\"],\"side\":\"TOP\"},\"type\":\"ConnectorPlacement.EquallySpacedRectSide\",\"uuid\":\"8a3cb844-269f-4d3f-b8ee-2af4584390c1\"},{\"content\":{\"connectorIds\":[\"In3\",\"In4\",\"In5\",\"In6\"],\"side\":\"BOTTOM\"},\"type\":\"ConnectorPlacement.EquallySpacedRectSide\",\"uuid\":\"ccc3bad4-265e-44f4-a8b0-aae769a28e60\"}]},\"type\":\"ConnectorPlacement.EquallySpacedConnector\",\"uuid\":\"9389ccda-4d08-49a8-9951-bd9019203c57\"}],\"packageUris\":[\"http://schema.mathworks.com/mf0/Connector/R2020b\"],\"version\":\"1.0\"}"
  q_opt computing : Subsystem
      settings: PortSchema="{\"entries\":[{\"content\":{\"sides\":[{\"content\":{\"connectorIds\":[\"In1\",\"In2\"]},\"type\":\"ConnectorPlacement.EquallySpacedRectSide\",\"uuid\":\"077e0174-8a2c-4f76-bac9-e91df836f5e1\"},{\"content\":{\"connectorIds\":[\"Out1\",\"In4\"],\"side\":\"RIGHT\"},\"type\":\"ConnectorPlacement.EquallySpacedRectSide\",\"uuid\":\"0e923535-8f32-4607-bd4a-42896d211835\"},{\"content\":{\"connectorIds\":[\"In3\"],\"side\":\"TOP\"},\"type\":\"ConnectorPlacement.EquallySpacedRectSide\",\"uuid\":\"91682e2a-1ae8-44b6-9458-d5d75f2c9b10\"},{\"content\":{\"side\":\"BOTTOM\"},\"type\":\"ConnectorPlacement.EquallySpacedRectSide\",\"uuid\":\"ebee2d10-c6a3-420b-a3da-5d4d259a0e4d\"}]},\"type\":\"ConnectorPlacement.EquallySpacedConnector\",\"uuid\":\"6651e596-192f-4f32-9855-13a8c081df01\"}],\"packageUris\":[\"http://schema.mathworks.com/mf0/Connector/R2020b\"],\"version\":\"1.0\"}"
  q_estimated : Outport
  wires:
  alpha 1/1 -> [alpha1]
  [B_b] -> B computing/3(Bb)
  S_b/1 -> [S_b]
  [B_N] -> B computing/4(BN)
  [S_N] -> B computing/2(SN)
  B computing/1(B) -> q_opt computing/4(B), S and Z matrix computing/1(B)
  [S_N] -> Subsystem/6(S_N)
  [B_b] -> Subsystem/3(B_b)
  [S_b] -> Subsystem/5(S_b)
  B_N/1 -> [B_N]
  S_N/1 -> [S_N]
  B_b/1 -> [B_b]
  [alpha1] -> B computing/5(alpha 1)
  [S_b] -> B computing/1(Sb)
  S and Z matrix computing/1(S) -> q_opt computing/1(S)
  [alpha2] -> B computing/6(alpha 2)
  alpha 2/1 -> [alpha2]
  S and Z matrix computing/2(Z) -> q_opt computing/2(Z)
  q_opt computing/1(q_opt) -> q_estimated/1
  [B_N] -> Subsystem/4(B_N)
  B computing/2(alpha1_normalised) -> Subsystem/2(alpha1_normalised)
  B computing/3(alpha2_normalised) -> Subsystem/1(alpha2_normalised)
  Subsystem/1(lambda_max) -> Scope/1, q_opt computing/3(lambda_max)

== system CubeSatTEST/OBC/Navigation1/Sequential Rotations Playground/Reference Rotator x ==
  S_N : Inport
  Action Port : ActionPort  ActionPortLabel=elseif((u1 == 1)&(u3==0))
  Demux : Demux  Outputs=3
  Gain : Gain  Gain=-1
  Gain1 : Gain  Gain=-1
  Gain2 : Gain
  Mux : Mux  Inputs=3
  Out1 : Outport
  wires:
  S_N/1 -> Demux/1
  Mux/1 -> Out1/1
  Gain2/1 -> Mux/1
  Gain/1 -> Mux/2
  Gain1/1 -> Mux/3
  Demux/1 -> Gain2/1
  Demux/2 -> Gain/1
  Demux/3 -> Gain1/1
